simulink model "PIDControl"  (R2018b)
settings: configuration reference "RPi_ControlRate" (kept outside this file)
InitFcn:
  | loadThrusterData
undefined symbols (not defined in the file or in its folder): DiscIntNeverNeededParam
libraries: simulink x12
settings Model: Creator=Andy  LastModifiedBy=barthal
settings ConfigSetRef: SourceLocation=Base Workspace

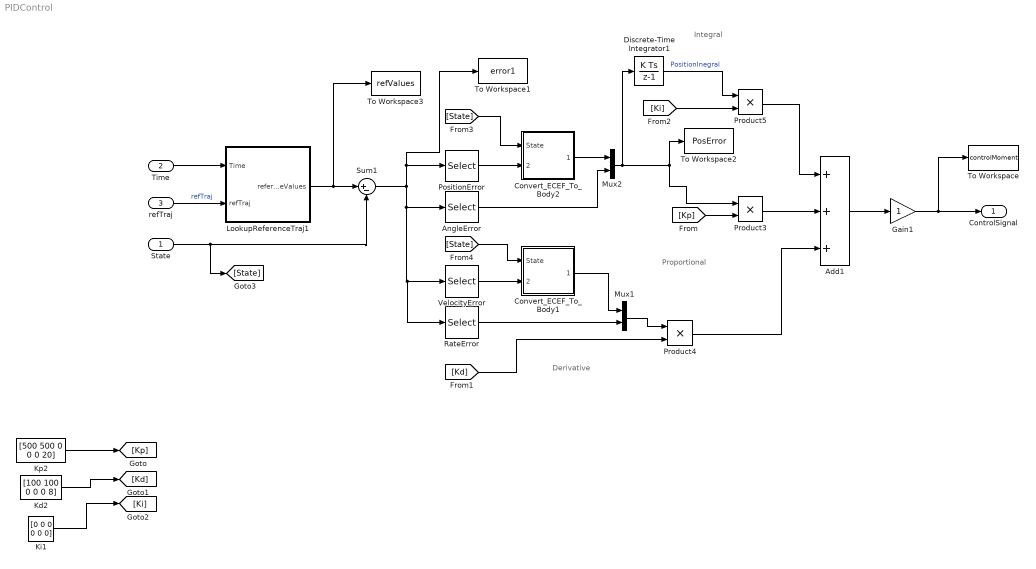
== system PIDControl ==
  note: Derivative
  note: Integral
  note: Proportional
  State : Inport  OutDataTypeStr=double
  Time : Inport  Port=2  OutDataTypeStr=double  PortDimensions=1
  refTraj : Inport  Port=3  OutDataTypeStr=double  PortDimensions=[5 13]
  Add1 : Sum  Inputs=+++
  AngleError : Selector  IndexOptions=Index vector (dialog)  Indices=[4:6]  OutputSizes=1
  Convert_ECEF_To_Body1 : Subsystem
  Convert_ECEF_To_Body2 : Subsystem
  Discrete-Time Integrator1 : DiscreteIntegrator  SampleTime=-1  ICPrevOutput=DiscIntNeverNeededParam  ICPrevScaledInput=DiscIntNeverNeededParam
  Gain1 : Gain
  Kd2 : Constant  Value=[100 100 0 0 0 8]
  Ki1 : Constant  Value=[0 0 0 0 0 0]
  Kp2 : Constant  Value=[500 500 0 0 0 20]
  LookupReferenceTraj1 : Subsystem
  Mux1 : Mux  Inputs=2
  Mux2 : Mux  Inputs=2
  PositionError : Selector  IndexOptions=Index vector (dialog)  Indices=[1:3]  OutputSizes=1
  Product3 : Product
  Product4 : Product
  Product5 : Product
  RateError : Selector  IndexOptions=Index vector (dialog)  Indices=[10:12]  OutputSizes=1
  Sum1 : Sum  Inputs=|+-
  To Workspace : ToWorkspace  VariableName=controlMoment  SaveFormat=Timeseries  SampleTime=-1
  To Workspace1 : ToWorkspace  VariableName=error1  SaveFormat=Timeseries  SampleTime=-1
  To Workspace2 : ToWorkspace  VariableName=PosError  SaveFormat=Timeseries  SampleTime=-1
  To Workspace3 : ToWorkspace  VariableName=refValues  SaveFormat=Timeseries  SampleTime=-1
  VelocityError : Selector  IndexOptions=Index vector (dialog)  Indices=[7:9]  OutputSizes=1
  ControlSignal : Outport  OutDataTypeStr=double
  wires:
  Add1/1 -> Gain1/1
  LookupReferenceTraj1/1(referenceValues) -> To Workspace3/1, Sum1/1
  Product4/1 -> Add1/3
  State/1 -> [State], Sum1/2
  [State] -> Convert_ECEF_To_Body2/1(State)
  [Kp] -> Product3/2
  Ki1/1 -> [Ki]
  Sum1/1 -> To Workspace1/1, PositionError/1, AngleError/1, RateError/1, VelocityError/1
  Kp2/1 -> [Kp]
  Convert_ECEF_To_Body2/1(Vec_Body) -> Mux2/1
  [Kd] -> Product4/2
  Gain1/1 -> To Workspace/1, ControlSignal/1
  [Ki] -> Product5/2
  Discrete-Time Integrator1/1 -> Product5/1  "PositionInegral"
  refTraj/1 -> LookupReferenceTraj1/2(refTraj)  "refTraj"
  Kd2/1 -> [Kd]
  VelocityError/1 -> Convert_ECEF_To_Body1/2(Vec_ECEF)
  [State] -> Convert_ECEF_To_Body1/1(State)
  Product5/1 -> Add1/1
  Product3/1 -> Add1/2
  PositionError/1 -> Convert_ECEF_To_Body2/2(Vec_ECEF)
  Time/1 -> LookupReferenceTraj1/1(Time)
  Convert_ECEF_To_Body1/1(Vec_Body) -> Mux1/1
  RateError/1 -> Mux1/2
  Mux1/1 -> Product4/1
  Mux2/1 -> Discrete-Time Integrator1/1, Product3/1, To Workspace2/1
  AngleError/1 -> Mux2/2

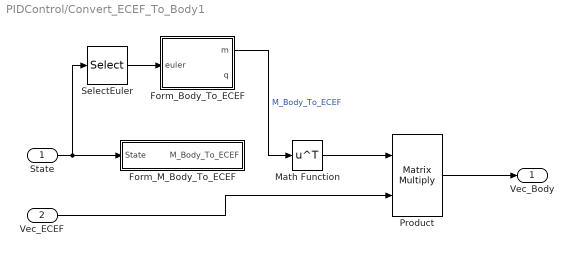
== system PIDControl/Convert_ECEF_To_Body1 ==
  State : Inport
  Vec_ECEF : Inport  Port=2  PortDimensions=3
  Form_Body_To_ECEF : MATLAB Function  TreatAsAtomicUnit=on
  Form_M_Body_To_ECEF : Subsystem
  Math Function : Math  Operator=transpose  SaturateOnIntegerOverflow=on
  Product : Product  Multiplication=Matrix(*)
  SelectEuler : Selector  InputPortWidth=12  IndexOptions=Index vector (dialog)  Indices=[4:6]  OutputSizes=1
  Vec_Body : Outport  PortDimensions=3
  wires:
  Math Function/1 -> Product/1
  Product/1 -> Vec_Body/1
  Vec_ECEF/1 -> Product/2
  State/1 -> SelectEuler/1, Form_M_Body_To_ECEF/1(State)
  SelectEuler/1 -> Form_Body_To_ECEF/1(euler)
  Form_Body_To_ECEF/1(m) -> Math Function/1  "M_Body_To_ECEF"

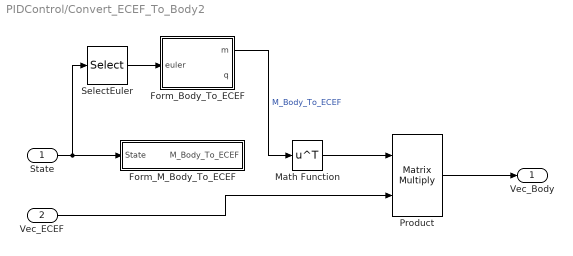
== system PIDControl/Convert_ECEF_To_Body2 ==
  State : Inport
  Vec_ECEF : Inport  Port=2  PortDimensions=3
  Form_Body_To_ECEF : MATLAB Function  TreatAsAtomicUnit=on
  Form_M_Body_To_ECEF : Subsystem
  Math Function : Math  Operator=transpose  SaturateOnIntegerOverflow=on
  Product : Product  Multiplication=Matrix(*)
  SelectEuler : Selector  InputPortWidth=12  IndexOptions=Index vector (dialog)  Indices=[4:6]  OutputSizes=1
  Vec_Body : Outport  PortDimensions=3
  wires:
  Math Function/1 -> Product/1
  Product/1 -> Vec_Body/1
  Vec_ECEF/1 -> Product/2
  State/1 -> SelectEuler/1, Form_M_Body_To_ECEF/1(State)
  SelectEuler/1 -> Form_Body_To_ECEF/1(euler)
  Form_Body_To_ECEF/1(m) -> Math Function/1  "M_Body_To_ECEF"

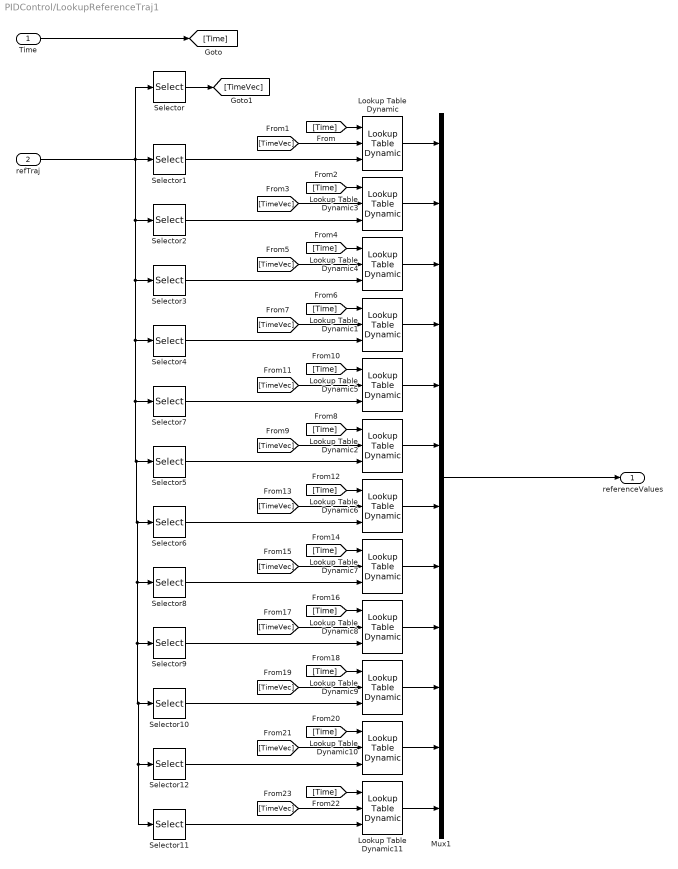
== system PIDControl/LookupReferenceTraj1 ==
  Time : Inport
  refTraj : Inport  Port=2
  Lookup Table Dynamic{,1..11} (12 alike) : simulink/Lookup Tables/Lookup Table Dynamic  LookUpMeth=Interpolation-Use End Values  OutDataType=fixdt('double')  OutScaling=[]  OutputDataTypeScalingMode=Specify via dialog  OutDataTypeStr=double  DoSatur=off
      settings: SourceProductName=Simulink
  Mux1 : Mux  Inputs=12
  Selector : Selector  NumberOfDimensions=2  InputPortWidth=3  IndexOptions=Select all,Index vector (dialog)  Indices=1,1  OutputSizes=1,1
  Selector1 : Selector  NumberOfDimensions=2  InputPortWidth=3  IndexOptions=Select all,Index vector (dialog)  Indices=1,2  OutputSizes=1,1
  Selector10 : Selector  NumberOfDimensions=2  InputPortWidth=3  IndexOptions=Select all,Index vector (dialog)  Indices=1,11  OutputSizes=1,1
  Selector11 : Selector  NumberOfDimensions=2  InputPortWidth=3  IndexOptions=Select all,Index vector (dialog)  Indices=1,13  OutputSizes=1,1
  Selector12 : Selector  NumberOfDimensions=2  InputPortWidth=3  IndexOptions=Select all,Index vector (dialog)  Indices=1,12  OutputSizes=1,1
  Selector2 : Selector  NumberOfDimensions=2  InputPortWidth=3  IndexOptions=Select all,Index vector (dialog)  Indices=1,3  OutputSizes=1,1
  Selector3 : Selector  NumberOfDimensions=2  InputPortWidth=3  IndexOptions=Select all,Index vector (dialog)  Indices=1,4  OutputSizes=1,1
  Selector4 : Selector  NumberOfDimensions=2  InputPortWidth=3  IndexOptions=Select all,Index vector (dialog)  Indices=1,5  OutputSizes=1,1
  Selector5 : Selector  NumberOfDimensions=2  InputPortWidth=3  IndexOptions=Select all,Index vector (dialog)  Indices=1,7  OutputSizes=1,1
  Selector6 : Selector  NumberOfDimensions=2  InputPortWidth=3  IndexOptions=Select all,Index vector (dialog)  Indices=1,8  OutputSizes=1,1
  Selector7 : Selector  NumberOfDimensions=2  InputPortWidth=3  IndexOptions=Select all,Index vector (dialog)  Indices=1,6  OutputSizes=1,1
  Selector8 : Selector  NumberOfDimensions=2  InputPortWidth=3  IndexOptions=Select all,Index vector (dialog)  Indices=1,9  OutputSizes=1,1
  Selector9 : Selector  NumberOfDimensions=2  InputPortWidth=3  IndexOptions=Select all,Index vector (dialog)  Indices=1,10  OutputSizes=1,1
  referenceValues : Outport
  wires:
  Lookup Table Dynamic2/1 -> Mux1/6
  Lookup Table Dynamic5/1 -> Mux1/5
  Lookup Table Dynamic1/1 -> Mux1/4
  Lookup Table Dynamic/1 -> Mux1/1
  Lookup Table Dynamic3/1 -> Mux1/2
  Lookup Table Dynamic4/1 -> Mux1/3
  Selector7/1 -> Lookup Table Dynamic5/3
  Selector5/1 -> Lookup Table Dynamic2/3
  [TimeVec] -> Lookup Table Dynamic2/2
  [Time] -> Lookup Table Dynamic4/1
  Selector3/1 -> Lookup Table Dynamic4/3
  [Time] -> Lookup Table Dynamic3/1
  Selector2/1 -> Lookup Table Dynamic3/3
  [TimeVec] -> Lookup Table Dynamic4/2
  [Time] -> Lookup Table Dynamic/1
  Selector1/1 -> Lookup Table Dynamic/3
  Mux1/1 -> referenceValues/1
  [TimeVec] -> Lookup Table Dynamic5/2
  Selector/1 -> [TimeVec]
  refTraj/1 -> Selector1/1, Selector/1, Selector2/1, Selector3/1, Selector4/1, Selector7/1, Selector11/1, Selector12/1, Selector10/1, Selector9/1, Selector8/1, Selector6/1, Selector5/1
  [Time] -> Lookup Table Dynamic5/1
  [TimeVec] -> Lookup Table Dynamic3/2
  [Time] -> Lookup Table Dynamic2/1
  [Time] -> Lookup Table Dynamic1/1
  Time/1 -> [Time]
  [TimeVec] -> Lookup Table Dynamic/2
  [TimeVec] -> Lookup Table Dynamic1/2
  Selector4/1 -> Lookup Table Dynamic1/3
  [TimeVec] -> Lookup Table Dynamic6/2
  [Time] -> Lookup Table Dynamic6/1
  Selector6/1 -> Lookup Table Dynamic6/3
  [TimeVec] -> Lookup Table Dynamic7/2
  [Time] -> Lookup Table Dynamic7/1
  Selector8/1 -> Lookup Table Dynamic7/3
  Selector10/1 -> Lookup Table Dynamic9/3
  [Time] -> Lookup Table Dynamic9/1
  [TimeVec] -> Lookup Table Dynamic9/2
  [TimeVec] -> Lookup Table Dynamic8/2
  [Time] -> Lookup Table Dynamic8/1
  Selector9/1 -> Lookup Table Dynamic8/3
  Selector11/1 -> Lookup Table Dynamic11/3
  [Time] -> Lookup Table Dynamic11/1
  [TimeVec] -> Lookup Table Dynamic11/2
  [TimeVec] -> Lookup Table Dynamic10/2
  [Time] -> Lookup Table Dynamic10/1
  Selector12/1 -> Lookup Table Dynamic10/3
  Lookup Table Dynamic11/1 -> Mux1/12
  Lookup Table Dynamic10/1 -> Mux1/11
  Lookup Table Dynamic9/1 -> Mux1/10
  Lookup Table Dynamic8/1 -> Mux1/9
  Lookup Table Dynamic7/1 -> Mux1/8
  Lookup Table Dynamic6/1 -> Mux1/7

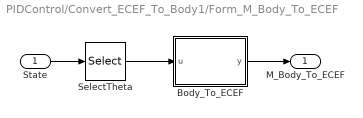
== system PIDControl/Convert_ECEF_To_Body1/Form_M_Body_To_ECEF ==
  State : Inport
  Body_To_ECEF : MATLAB Function  TreatAsAtomicUnit=on
  SelectTheta : Selector  InputPortWidth=12  IndexOptions=Index vector (dialog)  Indices=[6]  OutputSizes=1
  M_Body_To_ECEF : Outport
  wires:
  Body_To_ECEF/1(y) -> M_Body_To_ECEF/1
  SelectTheta/1 -> Body_To_ECEF/1(u)
  State/1 -> SelectTheta/1

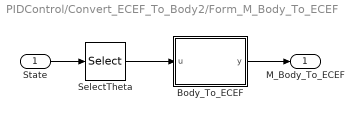
== system PIDControl/Convert_ECEF_To_Body2/Form_M_Body_To_ECEF ==
  State : Inport
  Body_To_ECEF : MATLAB Function  TreatAsAtomicUnit=on
  SelectTheta : Selector  InputPortWidth=12  IndexOptions=Index vector (dialog)  Indices=[6]  OutputSizes=1
  M_Body_To_ECEF : Outport
  wires:
  Body_To_ECEF/1(y) -> M_Body_To_ECEF/1
  SelectTheta/1 -> Body_To_ECEF/1(u)
  State/1 -> SelectTheta/1

== matlab function PIDControl/Convert_ECEF_To_Body1/Form_Body_To_ECEF ==
  data: euler input; m output; q output
function [m,q] = fcn(euler)

m = euler2mat(euler);
q = euler2quat(euler);

== matlab function PIDControl/Convert_ECEF_To_Body2/Form_Body_To_ECEF ==
  data: euler input; m output; q output
function [m,q] = fcn(euler)

m = euler2mat(euler);
q = euler2quat(euler);

== matlab function PIDControl/Convert_ECEF_To_Body1/Form_M_Body_To_ECEF/Body_To_ECEF ==
  data: u input; y output
function y = fcn(u)

y = [cos(u) -sin(u) 0; sin(u) cos(u) 0;0 0 1];

== matlab function PIDControl/Convert_ECEF_To_Body2/Form_M_Body_To_ECEF/Body_To_ECEF ==
  data: u input; y output
function y = fcn(u)

y = [cos(u) -sin(u) 0; sin(u) cos(u) 0;0 0 1];
